simulink model "BateriaLeds"  (R2023b)
settings: Solver=VariableStepAuto  StartTime=0.0  StopTime=Inf  RelTol=1e-3
libraries: simulink x4, arduinolib x3
settings Model: Creator=Andrés  LastModifiedBy=Andrés

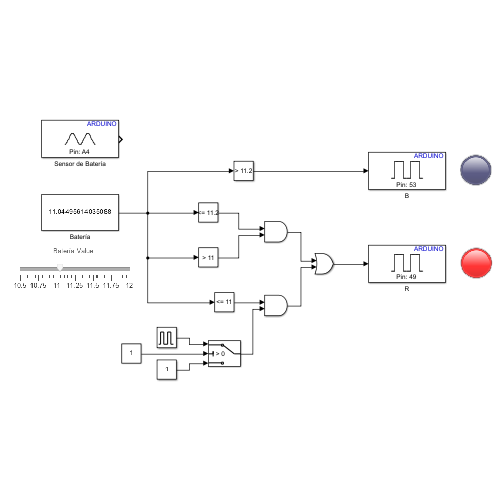
[thumbnail: Simulink's stored preview of the top-level diagram]
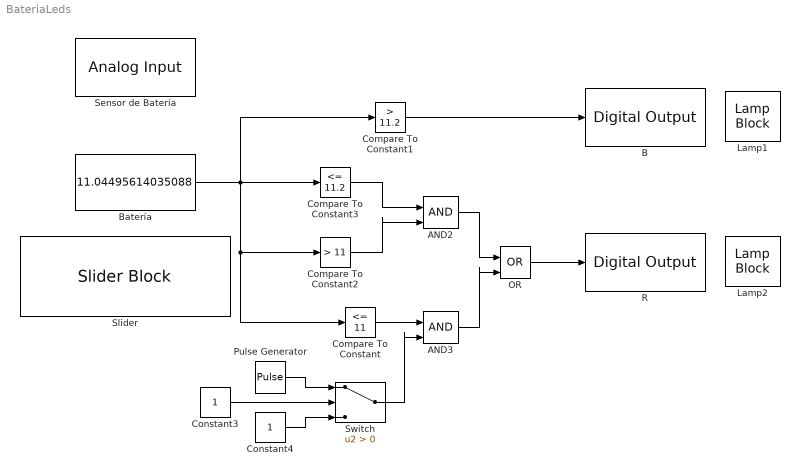
== system BateriaLeds ==
  AND2 : Logic  IconShape=distinctive  AllPortsSameDT=off  OutDataTypeStr=boolean
  AND3 : Logic  IconShape=distinctive  AllPortsSameDT=off  OutDataTypeStr=boolean
  B : arduinolib/Digital Output  pinNumber=53  Direction=output  blockPlatform=arduino
  Batería : Constant  Value=11.04495614035088
  Compare To Constant : simulink/Logic and Bit Operations/Compare To Constant  relop=<=  const=11  OutDataTypeStr=boolean
  Compare To Constant1 : simulink/Logic and Bit Operations/Compare To Constant  relop=>  const=11.2  OutDataTypeStr=boolean
  Compare To Constant2 : simulink/Logic and Bit Operations/Compare To Constant  relop=>  const=11  OutDataTypeStr=boolean
  Compare To Constant3 : simulink/Logic and Bit Operations/Compare To Constant  relop=<=  const=11.2  OutDataTypeStr=boolean
  Constant3 : Constant
  Constant4 : Constant
  Lamp1 : LampBlock  LabelPosition=Hide
  Lamp2 : LampBlock  LabelPosition=Hide
  OR : Logic  Operator=OR  IconShape=distinctive  AllPortsSameDT=off  OutDataTypeStr=boolean
  Pulse Generator : DiscretePulseGenerator  PulseType=Time based  Period=1  PulseWidth=50
  R : arduinolib/Digital Output  pinNumber=49  Direction=output  blockPlatform=arduino
  Sensor de Batería : arduinolib/Analog Input  pinNumber=4  ReadResultsOnly=off  ConversionTriggerSource=Software  ExternalTriggerType=uint32( 0 )  OutputDataType=uint16  EnableConversionCompleteNotify=off  EnableOuputStatus=off  SampleTime=-1  blockPlatform=arduino
  Slider : SliderBlock  ScaleMin=10.5  ScaleMax=12
  Switch : Switch  Criteria=u2 > Threshold  SaturateOnIntegerOverflow=off  InputSameDT=off
  wires:
  Pulse Generator/1 -> Switch/1
  Constant4/1 -> Switch/3
  Constant3/1 -> Switch/2
  Switch/1 -> AND3/2
  Compare To Constant/1 -> AND3/1
  Batería/1 -> Compare To Constant1/1, Compare To Constant2/1, Compare To Constant/1, Compare To Constant3/1
  Compare To Constant1/1 -> B/1
  Compare To Constant3/1 -> AND2/1
  Compare To Constant2/1 -> AND2/2
  OR/1 -> R/1
  AND3/1 -> OR/2
  AND2/1 -> OR/1
